simulink model "AUV_simulation_cmbined"  (R2024a)
settings: Solver=VariableStepAuto  StartTime=0.0  StopTime=10.0  RelTol=1e-3
model workspace (MAT data in the model file):
  T = 50
undefined symbols (not defined in the file): Acel_X, Acel_Y, Acel_Z, AUV, Cam_Left_Orientation, Cam_Left_Position, Cam_Right_Orientation, Cam_Right_Position, Gyro_X, Gyro_Y, Gyro_Z, Hydrophone_Bearing, Hydrophone_Distance, Leak_Detected, Pressure_Pa
libraries: nesl_utility x28, sm_lib x15, simulink x9
settings Model: Creator=adity  LastModifiedBy=adity

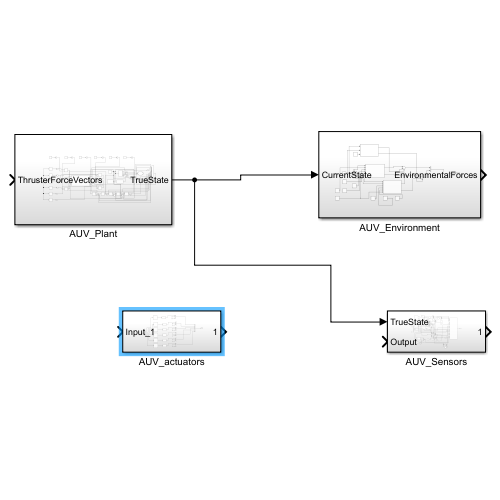
[thumbnail: Simulink's stored preview of the top-level diagram]
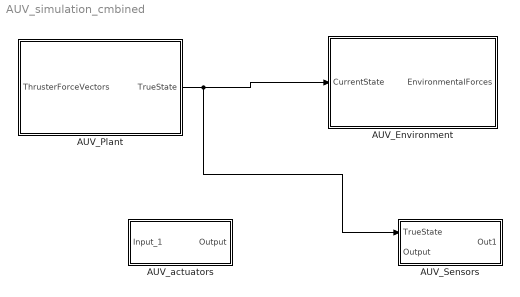
== system AUV_simulation_cmbined ==
  AUV_Environment : Subsystem
  AUV_Plant : Subsystem
  AUV_Sensors : Subsystem
  AUV_actuators : Subsystem
  wires:
  AUV_Plant/1(TrueState) -> AUV_Sensors/1(TrueState), AUV_Environment/1(CurrentState)

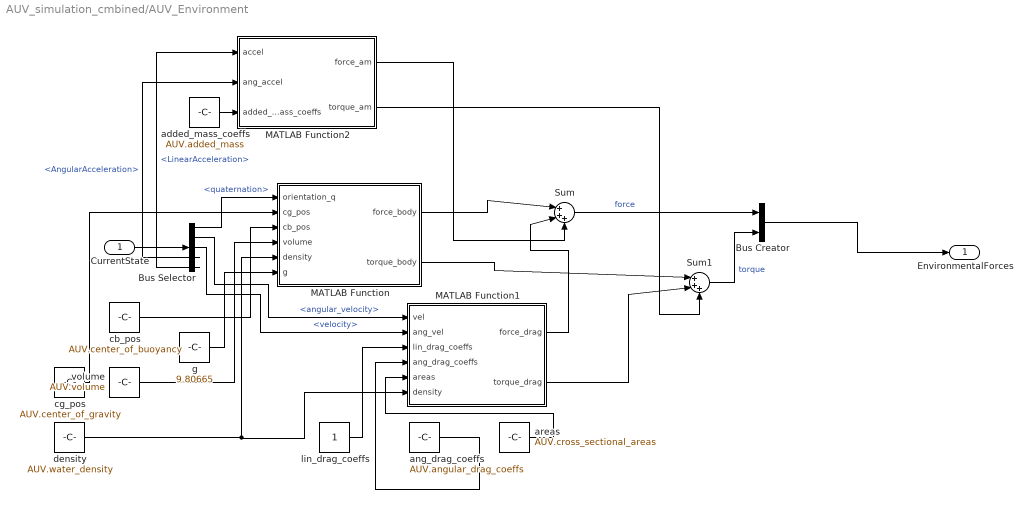
== system AUV_simulation_cmbined/AUV_Environment ==
  CurrentState : Inport
  Bus Creator : BusCreator  Inputs=2
  Bus Selector : BusSelector  OutputSignals=quaternation,angular_velocity,velocity,AngularAcceleration,LinearAcceleration
  MATLAB Function : MATLAB Function  TreatAsAtomicUnit=on
  MATLAB Function1 : MATLAB Function  TreatAsAtomicUnit=on
  MATLAB Function2 : MATLAB Function  TreatAsAtomicUnit=on
  Sum : Sum  Inputs=|+++
  Sum1 : Sum  Inputs=|+++
  added_mass_coeffs : Constant  Value=AUV.added_mass
  ang_drag_coeffs : Constant  Value=AUV.angular_drag_coeffs
  areas : Constant  Value=AUV.cross_sectional_areas
  cb_pos : Constant  Value=AUV.center_of_buoyancy
  cg_pos : Constant  Value=AUV.center_of_gravity
  density : Constant  Value=AUV.water_density
  g : Constant  Value=9.80665
  lin_drag_coeffs : Constant
  volume : Constant  Value=AUV.volume
  EnvironmentalForces : Outport
  wires:
  CurrentState/1 -> Bus Selector/1
  Bus Selector/1 -> MATLAB Function/1(orientation_q)  "<quaternation>"
  cg_pos/1 -> MATLAB Function/2(cg_pos)
  cb_pos/1 -> MATLAB Function/3(cb_pos)
  volume/1 -> MATLAB Function/4(volume)
  density/1 -> MATLAB Function/5(density), MATLAB Function1/6(density)
  g/1 -> MATLAB Function/6(g)
  Bus Selector/2 -> MATLAB Function1/1(vel)  "<angular_velocity>"
  Bus Selector/3 -> MATLAB Function1/2(ang_vel)  "<velocity>"
  areas/1 -> MATLAB Function1/5(areas)
  ang_drag_coeffs/1 -> MATLAB Function1/4(ang_drag_coeffs)
  lin_drag_coeffs/1 -> MATLAB Function1/3(lin_drag_coeffs)
  MATLAB Function/1(force_body) -> Sum/1
  MATLAB Function1/1(force_drag) -> Sum/2
  MATLAB Function/2(torque_body) -> Sum1/1
  MATLAB Function1/2(torque_drag) -> Sum1/2
  Sum/1 -> Bus Creator/1  "force"
  Sum1/1 -> Bus Creator/2  "torque"
  Bus Creator/1 -> EnvironmentalForces/1
  Bus Selector/4 -> MATLAB Function2/2(ang_accel)  "<AngularAcceleration>"
  Bus Selector/5 -> MATLAB Function2/1(accel)  "<LinearAcceleration>"
  added_mass_coeffs/1 -> MATLAB Function2/3(added_mass_coeffs)
  MATLAB Function2/2(torque_am) -> Sum1/3
  MATLAB Function2/1(force_am) -> Sum/3

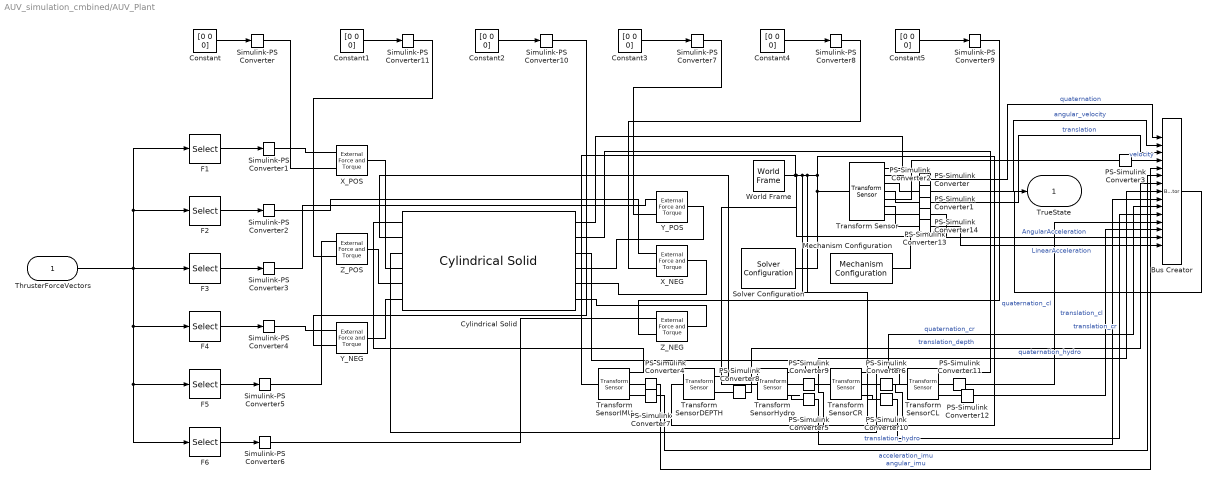
== system AUV_simulation_cmbined/AUV_Plant ==
  ThrusterForceVectors : Inport  PortDimensions=[6 3]
  Bus Creator : BusCreator  Inputs=15
  Constant{,1..5} (6 alike) : Constant  Value=[0 0 0]
  Cylindrical Solid : sm_lib/Body Elements/Cylindrical Solid  CylinderRadius=1  CylinderRadiusUnits=m  CylinderLength=1  CylinderLengthUnits=m  ExportEntireGeometry=off  InertiaType=Custom  BasedOnType=Density  Density=1000  DensityUnits=kg/m^3  Mass=AUV.mass  MassUnits=kg  CenterOfMass=AUV.center_of_gravity  CenterOfMassUnits=m  MomentsOfInertia=[AUV.inertia(1,1), AUV.inertia(2,2), AUV.inertia(3,3)]  MomentsOfInertiaUnits=kg*m^2  ProductsOfInertia=[AUV.inertia(2,3), AUV.inertia(1,3), AUV.inertia(1,2)]  ProductsOfInertiaUnits=kg*m^2  GraphicType=FromGeometry  MarkerShape=Sphere  MarkerSize=10  GraphicVisPropType=SimpleVisualProperties  GraphicDiffuseColor=[0.5 0.5 0.5]  GraphicOpacity=1  GraphicSpecularColor=[0.5 0.5 0.5 1.0]  GraphicAmbientColor=[0.15 0.15 0.15 1.0]  GraphicEmissiveColor=[0.0 0.0 0.0 1.0]  GraphicShininess=75  DoExposeReferenceFrame=on  SerializedFrames=<Frames><Frame><Id>Frame1</Id><Value><Name>IMU_Frame</Name><Origin><Source>ReferenceFrame</Source><FeatureName></FeatureName></Origin><PrimaryAxis><DefinedDirection>+Z</DefinedDirection><Source>ReferenceFrame</Source><SourceDirection>+Z</SourceDirection><FeatureName></FeatureName></PrimaryAxis><SecondaryAxis><DefinedDirection>+X</DefinedDirection><Source>ReferenceFrame</Source><SourceDirection>+X</SourceDirection><FeatureName></FeatureName></SecondaryAxis></Value></Frame><Frame><Id>Frame2</Id><Value><Name>DepthSensor_Frame</Name><Origin><Source>ReferenceFrame</Source><FeatureName></FeatureName></Origin><PrimaryAxis><DefinedDirection>+Z</DefinedDirection><Source>ReferenceFrame</Source><SourceDirection>+Z</SourceDirection><FeatureName></FeatureName></PrimaryAxis><SecondaryAxis><DefinedDirection>+X</DefinedDirection><Source>ReferenceFrame</Source><SourceDirection>+X</SourceDirection><FeatureName></FeatureName></SecondaryAxis></Value></Frame><Frame><Id>Frame3</Id><Value><Name>Camera_Left_Frame</Name><Origin><Source>ReferenceFrame</Source><FeatureName></FeatureName></Origin><PrimaryAxis><DefinedDirection>+Z</DefinedDirection><Source>ReferenceFrame</Source><SourceDirection>+Z</SourceDirection><FeatureName></FeatureName></PrimaryAxis><SecondaryAxis><DefinedDirection>+X</DefinedDirection><Source>ReferenceFrame</Source><SourceDirection>+X</SourceDirection><FeatureName></FeatureName></SecondaryAxis></Value></Frame><Frame><Id>Frame4</Id><Value><Name>Camera_Right_Frame</Name><Origin><Source>ReferenceFrame</Source><FeatureName></FeatureName></Origin><PrimaryAxis><DefinedDirection>+Z</DefinedDirection><Source>ReferenceFrame</Source><SourceDirection>+Z</SourceDirection><FeatureName></FeatureName></PrimaryAxis><SecondaryAxis><DefinedDirection>+X</DefinedDirection><Source>ReferenceFrame</Source><SourceDirection>+X</SourceDirection><FeatureName></FeatureName></SecondaryAxis></Value></Frame><Frame><Id>Frame5</Id><Value><Name>Hydrophone_Frame</Name><Origin><Source>ReferenceFrame</Source><FeatureName></FeatureName></Origin><PrimaryAxis><DefinedDirection>+Z</DefinedDirection><Source>ReferenceFrame</Source><SourceDirection>+Z</SourceDirection><FeatureName></FeatureName></PrimaryAxis><SecondaryAxis><DefinedDirection>+X</DefinedDirection><Source>ReferenceFrame</Source><SourceDirection>+X</SourceDirection><FeatureName></FeatureName></SecondaryAxis></Value></Frame><Frame><Id>Frame6</Id><Value><Name>Thruster_X_Pos</Name><Origin><Source>ReferenceFrame</Source><FeatureName></FeatureName></Origin><PrimaryAxis><DefinedDirection>+Z</DefinedDirection><Source>ReferenceFrame</Source><SourceDirection>+Z</SourceDirection><FeatureName></FeatureName></PrimaryAxis><SecondaryAxis><DefinedDirection>+X</DefinedDirection><Source>ReferenceFrame</Source><SourceDirection>+X</SourceDirection><FeatureName></FeatureName></SecondaryAxis></Value></Frame><Frame><Id>Frame7</Id><Value><Name>Thruster_Y_Pos</Name><Origin><Source>ReferenceFrame</Source><FeatureName></FeatureName></Origin><PrimaryAxis><DefinedDirection>+Z</DefinedDirection><Source>ReferenceFrame</Source><SourceDirection>+Z</SourceDirection><FeatureName></FeatureName></PrimaryAxis><SecondaryAxis><DefinedDirection>+X</DefinedDirection><Source>ReferenceFrame</Source><SourceDirection>+X</SourceDirection><FeatureName></FeatureName></SecondaryAxis></Value></Frame><Frame><Id>Frame8</Id><Value><Name>Thruster_Z_Pos</Name><Origin><Source>ReferenceFrame</Source><FeatureName></FeatureName></Origin><PrimaryAxis><DefinedDirection>+Z</DefinedDirection><Source>ReferenceFrame</Source><SourceDirection>+Z</SourceDirection><FeatureName></FeatureName></PrimaryAxis><SecondaryAxis><DefinedDirection>+X</DefinedDirection><Source>ReferenceFrame</Source><SourceDirection>+X</SourceDirection><FeatureName></FeatureName></SecondaryAxis></Value></Frame><Frame><Id>Frame9</Id><Value><Name>Thruster_X_Neg</Name><Origin><Source>ReferenceFrame</Source><FeatureName></FeatureName></Origin><PrimaryAxis><DefinedDirection>+Z</DefinedDirection><Source>ReferenceFrame</Source><SourceDirection>+Z</SourceDirection><FeatureName></FeatureName></PrimaryAxis><SecondaryAxis><DefinedDirection>+X</DefinedDirection><Source>ReferenceFrame</Source><SourceDirection>+X</SourceDirection><FeatureName></FeatureName></SecondaryAxis></Value></Frame><Frame><Id>Frame10</Id><Value><Name>Thruster_Y_Neg</Name><Origin><Source>ReferenceFrame</Source><FeatureName></FeatureName></Origin><PrimaryAxis><DefinedDirection>+Z</DefinedDirection><Source>ReferenceFrame</Source><SourceDirection>+Z</SourceDirection><FeatureName></FeatureName></PrimaryAxis><SecondaryAxis><DefinedDirection>+X</DefinedDirection><Source>ReferenceFrame</Source><SourceDirection>+X</SourceDirection><FeatureName></FeatureName></SecondaryAxis></Value></Frame><Frame><Id>Frame11</Id><Value><Name>Thruster_Z_Neg</Name><Origin><Source>ReferenceFrame</Source><FeatureName></FeatureName></Origin><PrimaryAxis><DefinedDirection>+Z</DefinedDirection><Source>ReferenceFrame</Source><SourceDirection>+Z</SourceDirection><FeatureName></FeatureName></PrimaryAxis><SecondaryAxis><DefinedDirection>+X</DefinedDirection><Source>ReferenceFrame</Source><SourceDirection>+X</SourceDirection><FeatureName></FeatureName></SecondaryAxis></Value></Frame></Frames>
  F1 : Selector  NumberOfDimensions=2  InputPortWidth=3  IndexOptions=Index vector (dialog),Select all  Indices=1,1  OutputSizes=1,1
  F2 : Selector  NumberOfDimensions=2  InputPortWidth=3  IndexOptions=Index vector (dialog),Select all  Indices=2,1  OutputSizes=1,1
  F3 : Selector  NumberOfDimensions=2  InputPortWidth=3  IndexOptions=Index vector (dialog),Select all  Indices=3,1  OutputSizes=1,1
  F4 : Selector  NumberOfDimensions=2  InputPortWidth=3  IndexOptions=Index vector (dialog),Select all  Indices=4,1  OutputSizes=1,1
  F5 : Selector  NumberOfDimensions=2  InputPortWidth=3  IndexOptions=Index vector (dialog),Select all  Indices=5,1  OutputSizes=1,1
  F6 : Selector  NumberOfDimensions=2  InputPortWidth=3  IndexOptions=Index vector (dialog),Select all  Indices=6,1  OutputSizes=1,1
  Mechanism Configuration : sm_lib/Utilities/Mechanism Configuration  UniformGravity=Constant  GravityVector=[0 0 9.80665]  GravityVectorUnits=m/s^2  LinearizationDelta=0.001  JointModeTransitionNonlinearIterations=2
  PS-Simulink Converter{,1..14} (15 alike) : nesl_utility/PS-Simulink Converter  PhysicalDomain=network_engine_domain  SubClassName=ps_output  LeftPortType=input  RightPortType=output  PseudoPeriodic=off  Frequencies=[]  VectorFormat=inherit  Unit=inherit  AffineConversion=off
  Simulink-PS Converter{,1..11} (12 alike) : nesl_utility/Simulink-PS Converter  PhysicalDomain=network_engine_domain  SubClassName=ps_input  LeftPortType=input  RightPortType=output  PseudoPeriodic=off  Frequencies=[]  NoiseDistribution=none  NoiseParameters=[]  Unit=1  AffineConversion=off  FilteringAndDerivatives=provide  SimscapeFilterOrder=1  InputFilterTimeConstant=0.001  UdotUserProvided=0
  Solver Configuration : nesl_utility/Solver Configuration  PhysicalDomain=network_engine_domain  SubClassName=solver  LeftPortType=input  RightPortType=generic  Tones=[]  Harmonics=[]  SimulateNoise=off  Profile=off  UseLocalSampling=off  EnableSwitchedLinearOptims=on  FrequencyDomain=off  UseCCode=off  RelTol=0.001  AbsTol=0.001  MinStep=1e-09  ToWorkspace=off  RevertToSquareIcSolve=off  NumHomotopyIterations=100  PhasorMode=off  PhasorModeNumHarmonics=1  ConsistencySolver=NEWTON_XTOL_AFTER_FTOL  IndexReductionMethod=DerivativeReplacement  DoDC=off  ResidualTolerance=1e-09  ConsistencyTolSource=GLOBAL  ConsistencyAbsTol=0.001  ConsistencyRelTol=0.001  ConsistencyTolFactor=0.001  UseLocalSolver=off  LocalSolverChoice=NE_BACKWARD_EULER_ADVANCER  ResolveIndetEquations=on  FunctionEvalNumThread=1  LocalSolverSampleTime=0.001  DoFixedCost=off  MaxNonlinIter=3  MaxModeIter=2  ComputeImpulses=off  ImpulseIterations=2  LinearAlgebra=auto  LinearAlgebraNumThread=0  EquationFormulation=NE_TIME_EF  DelaysMemoryBudget=1024  AutomaticFiltering=on  FilteringTimeConstant=0.001  PartitionStorageMethod=AS_NEEDED  PartitionMemoryBudget=1024  PartitionMethod=ROBUST  MultibodyUseLocalSolver=off  MultibodyLocalSolverChoice=ODE1  MultibodyLocalSolverSampleTime=0.001
  Transform Sensor : sm_lib/Frames and Transforms/Transform Sensor  MeasurementFrame=World  RotationSequence=XYX  SenseAngle=off  SenseAxis=off  SenseQ=on  SenseR=off  SenseRotationSequence=off  SenseOmegaX=off  SenseOmegaY=off  SenseOmegaZ=off  SenseOmega=on  SenseQDot=off  SenseRDot=off  SenseRotationSequenceDot=off  SenseAlphaX=off  SenseAlphaY=off  SenseAlphaZ=off  SenseAlpha=on  SenseQDDot=off  SenseRDDot=off  SenseX=off  SenseY=off  SenseZ=off  SenseXYZ=on  SenseRad=off  SenseAzim=off  SenseDist=off  SenseInc=off  SenseXDot=off  SenseYDot=off  SenseZDot=off  SenseXYZDot=on  SenseRadDot=off  SenseAzimDot=off  SenseDistDot=off  SenseIncDot=off  SenseXDDot=off  SenseYDDot=off  SenseZDDot=off  SenseXYZDDot=on  SenseRadDDot=off  SenseAzimDDot=off  SenseDistDDot=off  SenseIncDDot=off
  Transform SensorCL : sm_lib/Frames and Transforms/Transform Sensor  MeasurementFrame=World  RotationSequence=XYX  SenseAngle=off  SenseAxis=off  SenseQ=on  SenseR=off  SenseRotationSequence=off  SenseOmegaX=off  SenseOmegaY=off  SenseOmegaZ=off  SenseOmega=off  SenseQDot=off  SenseRDot=off  SenseRotationSequenceDot=off  SenseAlphaX=off  SenseAlphaY=off  SenseAlphaZ=off  SenseAlpha=off  SenseQDDot=off  SenseRDDot=off  SenseX=off  SenseY=off  SenseZ=off  SenseXYZ=on  SenseRad=off  SenseAzim=off  SenseDist=off  SenseInc=off  SenseXDot=off  SenseYDot=off  SenseZDot=off  SenseXYZDot=off  SenseRadDot=off  SenseAzimDot=off  SenseDistDot=off  SenseIncDot=off  SenseXDDot=off  SenseYDDot=off  SenseZDDot=off  SenseXYZDDot=off  SenseRadDDot=off  SenseAzimDDot=off  SenseDistDDot=off  SenseIncDDot=off
  Transform SensorCR : sm_lib/Frames and Transforms/Transform Sensor  MeasurementFrame=World  RotationSequence=XYX  SenseAngle=off  SenseAxis=off  SenseQ=on  SenseR=off  SenseRotationSequence=off  SenseOmegaX=off  SenseOmegaY=off  SenseOmegaZ=off  SenseOmega=off  SenseQDot=off  SenseRDot=off  SenseRotationSequenceDot=off  SenseAlphaX=off  SenseAlphaY=off  SenseAlphaZ=off  SenseAlpha=off  SenseQDDot=off  SenseRDDot=off  SenseX=off  SenseY=off  SenseZ=off  SenseXYZ=on  SenseRad=off  SenseAzim=off  SenseDist=off  SenseInc=off  SenseXDot=off  SenseYDot=off  SenseZDot=off  SenseXYZDot=off  SenseRadDot=off  SenseAzimDot=off  SenseDistDot=off  SenseIncDot=off  SenseXDDot=off  SenseYDDot=off  SenseZDDot=off  SenseXYZDDot=off  SenseRadDDot=off  SenseAzimDDot=off  SenseDistDDot=off  SenseIncDDot=off
  Transform SensorDEPTH : sm_lib/Frames and Transforms/Transform Sensor  MeasurementFrame=World  RotationSequence=XYX  SenseAngle=off  SenseAxis=off  SenseQ=off  SenseR=off  SenseRotationSequence=off  SenseOmegaX=off  SenseOmegaY=off  SenseOmegaZ=off  SenseOmega=off  SenseQDot=off  SenseRDot=off  SenseRotationSequenceDot=off  SenseAlphaX=off  SenseAlphaY=off  SenseAlphaZ=off  SenseAlpha=off  SenseQDDot=off  SenseRDDot=off  SenseX=off  SenseY=off  SenseZ=off  SenseXYZ=on  SenseRad=off  SenseAzim=off  SenseDist=off  SenseInc=off  SenseXDot=off  SenseYDot=off  SenseZDot=off  SenseXYZDot=off  SenseRadDot=off  SenseAzimDot=off  SenseDistDot=off  SenseIncDot=off  SenseXDDot=off  SenseYDDot=off  SenseZDDot=off  SenseXYZDDot=off  SenseRadDDot=off  SenseAzimDDot=off  SenseDistDDot=off  SenseIncDDot=off
  Transform SensorHydro : sm_lib/Frames and Transforms/Transform Sensor  MeasurementFrame=World  RotationSequence=XYX  SenseAngle=off  SenseAxis=off  SenseQ=on  SenseR=off  SenseRotationSequence=off  SenseOmegaX=off  SenseOmegaY=off  SenseOmegaZ=off  SenseOmega=off  SenseQDot=off  SenseRDot=off  SenseRotationSequenceDot=off  SenseAlphaX=off  SenseAlphaY=off  SenseAlphaZ=off  SenseAlpha=off  SenseQDDot=off  SenseRDDot=off  SenseX=off  SenseY=off  SenseZ=off  SenseXYZ=on  SenseRad=off  SenseAzim=off  SenseDist=off  SenseInc=off  SenseXDot=off  SenseYDot=off  SenseZDot=off  SenseXYZDot=off  SenseRadDot=off  SenseAzimDot=off  SenseDistDot=off  SenseIncDot=off  SenseXDDot=off  SenseYDDot=off  SenseZDDot=off  SenseXYZDDot=off  SenseRadDDot=off  SenseAzimDDot=off  SenseDistDDot=off  SenseIncDDot=off
  Transform SensorIMU : sm_lib/Frames and Transforms/Transform Sensor  MeasurementFrame=World  RotationSequence=XYX  SenseAngle=off  SenseAxis=off  SenseQ=off  SenseR=off  SenseRotationSequence=off  SenseOmegaX=off  SenseOmegaY=off  SenseOmegaZ=off  SenseOmega=on  SenseQDot=off  SenseRDot=off  SenseRotationSequenceDot=off  SenseAlphaX=off  SenseAlphaY=off  SenseAlphaZ=off  SenseAlpha=off  SenseQDDot=off  SenseRDDot=off  SenseX=off  SenseY=off  SenseZ=off  SenseXYZ=off  SenseRad=off  SenseAzim=off  SenseDist=off  SenseInc=off  SenseXDot=off  SenseYDot=off  SenseZDot=off  SenseXYZDot=off  SenseRadDot=off  SenseAzimDot=off  SenseDistDot=off  SenseIncDot=off  SenseXDDot=off  SenseYDDot=off  SenseZDDot=off  SenseXYZDDot=on  SenseRadDDot=off  SenseAzimDDot=off  SenseDistDDot=off  SenseIncDDot=off
  World Frame : sm_lib/Frames and Transforms/World Frame
  X_NEG : sm_lib/Forces and Torques/External Force and Torque  EnableForceX=off  EnableForceY=off  EnableForceZ=off  EnableForce=on  ForceResolutionFrame=AttachedFrame  EnableTorqueX=off  EnableTorqueY=off  EnableTorqueZ=off  EnableTorque=on  TorqueResolutionFrame=AttachedFrame
  X_POS : sm_lib/Forces and Torques/External Force and Torque  EnableForceX=off  EnableForceY=off  EnableForceZ=off  EnableForce=on  ForceResolutionFrame=AttachedFrame  EnableTorqueX=off  EnableTorqueY=off  EnableTorqueZ=off  EnableTorque=on  TorqueResolutionFrame=AttachedFrame
  Y_NEG : sm_lib/Forces and Torques/External Force and Torque  EnableForceX=off  EnableForceY=off  EnableForceZ=off  EnableForce=on  ForceResolutionFrame=AttachedFrame  EnableTorqueX=off  EnableTorqueY=off  EnableTorqueZ=off  EnableTorque=on  TorqueResolutionFrame=AttachedFrame
  Y_POS : sm_lib/Forces and Torques/External Force and Torque  EnableForceX=off  EnableForceY=off  EnableForceZ=off  EnableForce=on  ForceResolutionFrame=AttachedFrame  EnableTorqueX=off  EnableTorqueY=off  EnableTorqueZ=off  EnableTorque=on  TorqueResolutionFrame=AttachedFrame
  Z_NEG : sm_lib/Forces and Torques/External Force and Torque  EnableForceX=off  EnableForceY=off  EnableForceZ=off  EnableForce=on  ForceResolutionFrame=AttachedFrame  EnableTorqueX=off  EnableTorqueY=off  EnableTorqueZ=off  EnableTorque=on  TorqueResolutionFrame=AttachedFrame
  Z_POS : sm_lib/Forces and Torques/External Force and Torque  EnableForceX=off  EnableForceY=off  EnableForceZ=off  EnableForce=on  ForceResolutionFrame=AttachedFrame  EnableTorqueX=off  EnableTorqueY=off  EnableTorqueZ=off  EnableTorque=on  TorqueResolutionFrame=AttachedFrame
  TrueState : Outport
  wires:
  ThrusterForceVectors/1 -> F6/1, F5/1, F4/1, F3/1, F2/1, F1/1
  F1/1 -> Simulink-PS Converter1/1
  F2/1 -> Simulink-PS Converter2/1
  F3/1 -> Simulink-PS Converter3/1
  F4/1 -> Simulink-PS Converter4/1
  F5/1 -> Simulink-PS Converter5/1
  F6/1 -> Simulink-PS Converter6/1
  Constant/1 -> Simulink-PS Converter/1
  Constant1/1 -> Simulink-PS Converter11/1
  Constant2/1 -> Simulink-PS Converter10/1
  Constant3/1 -> Simulink-PS Converter7/1
  Constant4/1 -> Simulink-PS Converter8/1
  Constant5/1 -> Simulink-PS Converter9/1
  Bus Creator/1 -> TrueState/1
  PS-Simulink Converter/1 -> Bus Creator/1  "quaternation"
  PS-Simulink Converter2/1 -> Bus Creator/2  "angular_velocity"
  PS-Simulink Converter1/1 -> Bus Creator/3  "translation"
  PS-Simulink Converter3/1 -> Bus Creator/4  "velocity"
  PS-Simulink Converter4/1 -> Bus Creator/5  "angular_imu"
  PS-Simulink Converter7/1 -> Bus Creator/6  "acceleration_imu"
  PS-Simulink Converter8/1 -> Bus Creator/7  "translation_depth"
  PS-Simulink Converter9/1 -> Bus Creator/8  "quaternation_hydro"
  PS-Simulink Converter5/1 -> Bus Creator/9  "translation_hydro"
  PS-Simulink Converter6/1 -> Bus Creator/10  "quaternation_cr"
  PS-Simulink Converter10/1 -> Bus Creator/11  "translation_cr"
  PS-Simulink Converter11/1 -> Bus Creator/12  "quaternation_cl"
  PS-Simulink Converter12/1 -> Bus Creator/13  "translation_cl"
  PS-Simulink Converter14/1 -> Bus Creator/15  "LinearAcceleration"
  PS-Simulink Converter13/1 -> Bus Creator/14  "AngularAcceleration"
  connections:
  Cylindrical Solid/LConn4 -- X_POS/RConn1
  X_NEG/RConn1 -- Cylindrical Solid/RConn5
  Y_POS/RConn1 -- Cylindrical Solid/RConn4
  Z_NEG/RConn1 -- Cylindrical Solid/RConn6
  Y_NEG/RConn1 -- Cylindrical Solid/LConn6
  Z_POS/RConn1 -- Cylindrical Solid/LConn5
  Simulink-PS Converter1/RConn1 -- X_POS/LConn1
  Simulink-PS Converter2/RConn1 -- X_NEG/LConn1
  Simulink-PS Converter3/RConn1 -- Y_POS/LConn1
  Y_NEG/LConn1 -- Simulink-PS Converter4/RConn1
  Simulink-PS Converter5/RConn1 -- Z_POS/LConn1
  Simulink-PS Converter6/RConn1 -- Z_NEG/LConn1
  Simulink-PS Converter/RConn1 -- X_POS/LConn2
  Simulink-PS Converter11/RConn1 -- Z_POS/LConn2
  Simulink-PS Converter10/RConn1 -- Y_NEG/LConn2
  Simulink-PS Converter9/RConn1 -- Z_NEG/LConn2
  Simulink-PS Converter8/RConn1 -- X_NEG/LConn2
  Simulink-PS Converter7/RConn1 -- Y_POS/LConn2
  World Frame/RConn1 -- Transform SensorIMU/LConn1 -- Transform SensorHydro/LConn1 -- Mechanism Configuration/RConn1 -- Transform SensorDEPTH/LConn1 -- Transform SensorCL/LConn1 -- Transform SensorCR/LConn1 -- Solver Configuration/RConn1 -- Transform Sensor/LConn1
  Transform Sensor/RConn1 -- Cylindrical Solid/RConn1
  Transform Sensor/RConn2 -- PS-Simulink Converter/LConn1
  PS-Simulink Converter2/LConn1 -- Transform Sensor/RConn3
  PS-Simulink Converter1/LConn1 -- Transform Sensor/RConn4
  PS-Simulink Converter3/LConn1 -- Transform Sensor/RConn5
  Cylindrical Solid/LConn1 -- Transform SensorIMU/RConn1
  Transform SensorDEPTH/RConn1 -- Cylindrical Solid/LConn2
  Transform SensorHydro/RConn1 -- Cylindrical Solid/RConn3
  Cylindrical Solid/LConn3 -- Transform SensorCR/RConn1
  Transform SensorCL/RConn1 -- Cylindrical Solid/RConn2
  PS-Simulink Converter4/LConn1 -- Transform SensorIMU/RConn2
  PS-Simulink Converter7/LConn1 -- Transform SensorIMU/RConn3
  PS-Simulink Converter8/LConn1 -- Transform SensorDEPTH/RConn2
  PS-Simulink Converter6/LConn1 -- Transform SensorCR/RConn2
  Transform SensorHydro/RConn2 -- PS-Simulink Converter9/LConn1
  Transform SensorHydro/RConn3 -- PS-Simulink Converter5/LConn1
  PS-Simulink Converter10/LConn1 -- Transform SensorCR/RConn3
  PS-Simulink Converter12/LConn1 -- Transform SensorCL/RConn3
  PS-Simulink Converter11/LConn1 -- Transform SensorCL/RConn2
  PS-Simulink Converter13/LConn1 -- Transform Sensor/RConn6
  Transform Sensor/RConn7 -- PS-Simulink Converter14/LConn1

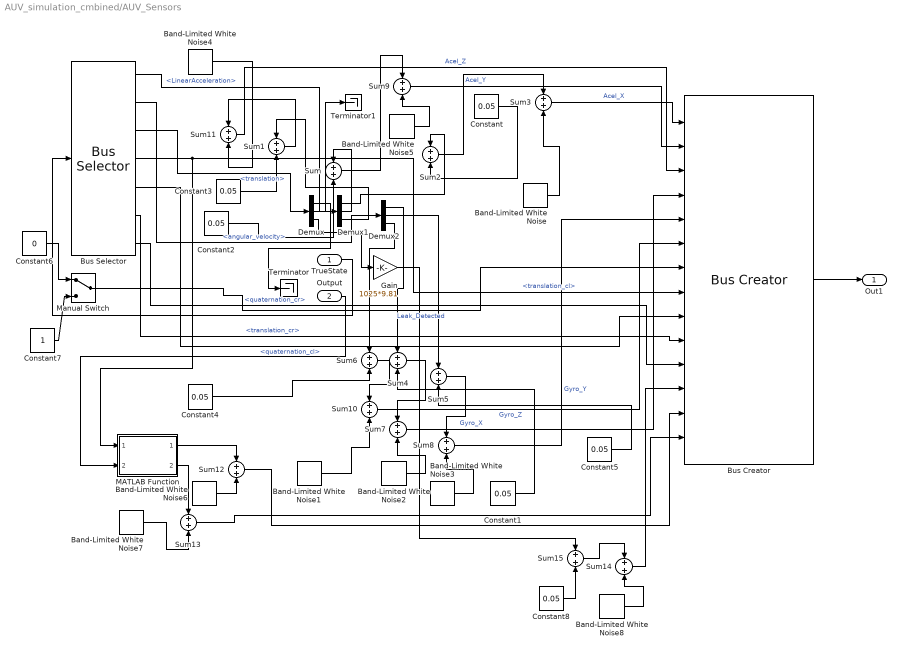
== system AUV_simulation_cmbined/AUV_Sensors ==
  TrueState : Inport
  Output : Inport  Port=2
  Band-Limited White Noise{,1..8} (9 alike) : simulink/Sources/Band-Limited White Noise  Cov=[0.1]  Ts=0.1  seed=[23341]
  Bus Creator : BusCreator  Inputs=Acel_X,Acel_Y,Acel_Z,Gyro_X,Gyro_Y,Gyro_Z,Leak_Detected,Cam_Left_Position,Cam_Left_Orientation,Cam_Right_Position,Cam_Right_Orientation,Pressure_Pa,Hydrophone_Distance,Hydrophone_Bearing
  Bus Selector : BusSelector  OutputSignals=LinearAcceleration,angular_velocity,translation,translation_cl,quaternation_cl,translation_cr,quaternation_cr
  Constant{,1..5,8} (7 alike) : Constant  Value=0.05
  Constant6 : Constant  Value=0
  Constant7 : Constant
  Demux : Demux  Outputs=3
  Demux1 : Demux  Outputs=3
  Demux2 : Demux  Outputs=3
  Gain : Gain  Gain=1025*9.81
  MATLAB Function : MATLAB Function  TreatAsAtomicUnit=on
  Manual Switch : ManualSwitch
  Sum{,1..15} (16 alike) : Sum
  Terminator : Terminator
  Terminator1 : Terminator
  Out1 : Outport
  wires:
  TrueState/1 -> Bus Selector/1
  Bus Creator/1 -> Out1/1
  Bus Selector/3 -> Demux/1  "<translation>"
  Bus Selector/1 -> Demux1/1  "<LinearAcceleration>"
  Bus Selector/2 -> Demux2/1  "<angular_velocity>"
  Demux/3 -> Gain/1
  Demux1/1 -> Sum2/1
  Constant/1 -> Sum2/2
  Sum2/1 -> Sum3/1
  Band-Limited White Noise/1 -> Sum3/2
  Demux1/2 -> Sum/1
  Demux1/3 -> Sum1/1
  Demux2/1 -> Sum4/1
  Demux2/2 -> Sum5/1
  Demux2/3 -> Sum6/1
  Constant4/1 -> Sum6/2
  Constant3/1 -> Sum1/2
  Constant2/1 -> Sum/2
  Constant1/1 -> Sum4/2
  Constant5/1 -> Sum5/2
  Sum1/1 -> Sum11/1
  Sum/1 -> Sum9/1
  Sum6/1 -> Sum10/1
  Sum4/1 -> Sum7/1
  Sum5/1 -> Sum8/1
  Band-Limited White Noise1/1 -> Sum10/2
  Band-Limited White Noise2/1 -> Sum7/2
  Band-Limited White Noise3/1 -> Sum8/2
  Band-Limited White Noise4/1 -> Sum11/2
  Band-Limited White Noise5/1 -> Sum9/2
  Sum3/1 -> Bus Creator/1  "Acel_X"
  Sum9/1 -> Bus Creator/2  "Acel_Y"
  Sum11/1 -> Bus Creator/3  "Acel_Z"
  Sum7/1 -> Bus Creator/4  "Gyro_X"
  Sum8/1 -> Bus Creator/5  "Gyro_Y"
  Sum10/1 -> Bus Creator/6  "Gyro_Z"
  Constant6/1 -> Manual Switch/1
  Constant7/1 -> Manual Switch/2
  Manual Switch/1 -> Bus Creator/7  "Leak_Detected"
  Bus Selector/4 -> Bus Creator/8, MATLAB Function/1(auv_pos)  "<translation_cl>"
  Bus Selector/5 -> Bus Creator/9  "<quaternation_cl>"
  Bus Selector/6 -> Bus Creator/10  "<translation_cr>"
  Bus Selector/7 -> Bus Creator/11  "<quaternation_cr>"
  Output/1 -> MATLAB Function/2(beacon_pos)
  MATLAB Function/1(distance) -> Sum12/1
  Band-Limited White Noise6/1 -> Sum12/2
  Band-Limited White Noise7/1 -> Sum13/2
  MATLAB Function/2(bearing) -> Sum13/1
  Sum12/1 -> Bus Creator/13
  Sum13/1 -> Bus Creator/14
  Gain/1 -> Sum15/1
  Constant8/1 -> Sum15/2
  Sum15/1 -> Sum14/1
  Band-Limited White Noise8/1 -> Sum14/2
  Sum14/1 -> Bus Creator/12
  Demux/1 -> Terminator/1
  Demux/2 -> Terminator1/1

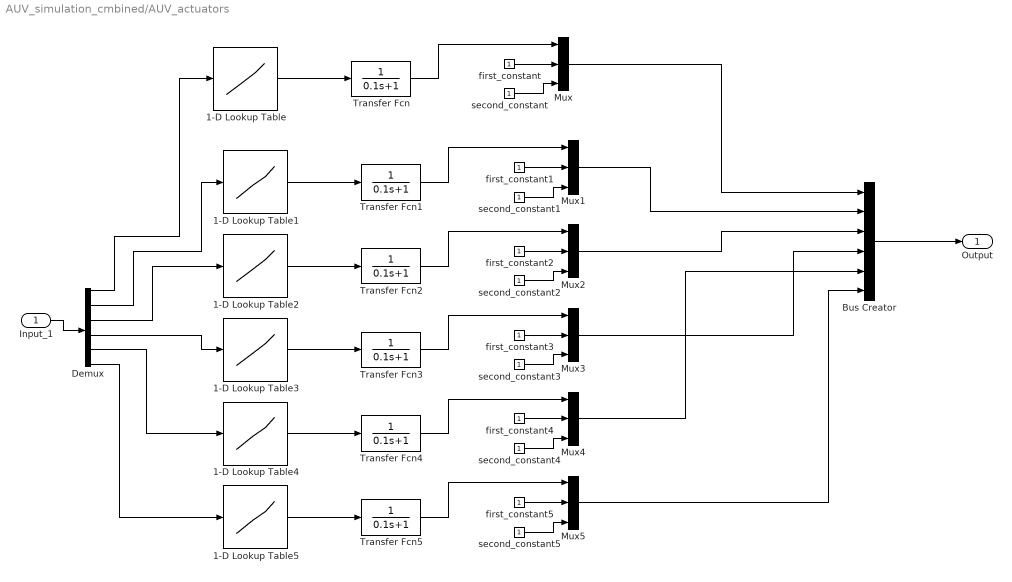
== system AUV_simulation_cmbined/AUV_actuators ==
  Input_1 : Inport
  1-D Lookup Table{,1..5} (6 alike) : Lookup_n-D  NumberOfTableDimensions=1  BreakpointsForDimension1=[-1,-0.1,0,0.1,1]  Table=[-40,-1,0,1,50]  InternalRulePriority=Speed  RndMeth=Simplest
  Bus Creator : BusCreator  Inputs=6
  Demux : Demux  Outputs=6
  Mux{,1..5} (6 alike) : Mux  Inputs=3
  Transfer Fcn{,1..5} (6 alike) : TransferFcn  Denominator=[0.1 1]
  first_constant{,1..5} (6 alike) : Constant
  second_constant{,1..5} (6 alike) : Constant
  Output : Outport
  wires:
  Demux/1 -> 1-D Lookup Table/1
  1-D Lookup Table/1 -> Transfer Fcn/1
  Transfer Fcn/1 -> Mux/1
  first_constant/1 -> Mux/2
  second_constant/1 -> Mux/3
  first_constant1/1 -> Mux1/2
  1-D Lookup Table1/1 -> Transfer Fcn1/1
  second_constant1/1 -> Mux1/3
  Demux/2 -> 1-D Lookup Table1/1
  Transfer Fcn1/1 -> Mux1/1
  Transfer Fcn2/1 -> Mux2/1
  second_constant2/1 -> Mux2/3
  first_constant2/1 -> Mux2/2
  1-D Lookup Table2/1 -> Transfer Fcn2/1
  Demux/3 -> 1-D Lookup Table2/1
  Transfer Fcn3/1 -> Mux3/1
  second_constant3/1 -> Mux3/3
  first_constant3/1 -> Mux3/2
  1-D Lookup Table3/1 -> Transfer Fcn3/1
  Demux/4 -> 1-D Lookup Table3/1
  Transfer Fcn4/1 -> Mux4/1
  second_constant4/1 -> Mux4/3
  first_constant4/1 -> Mux4/2
  1-D Lookup Table4/1 -> Transfer Fcn4/1
  Demux/5 -> 1-D Lookup Table4/1
  Transfer Fcn5/1 -> Mux5/1
  second_constant5/1 -> Mux5/3
  first_constant5/1 -> Mux5/2
  1-D Lookup Table5/1 -> Transfer Fcn5/1
  Demux/6 -> 1-D Lookup Table5/1
  Mux/1 -> Bus Creator/1
  Mux1/1 -> Bus Creator/2
  Mux2/1 -> Bus Creator/3
  Mux3/1 -> Bus Creator/4
  Mux4/1 -> Bus Creator/5
  Mux5/1 -> Bus Creator/6
  Input_1/1 -> Demux/1
  Bus Creator/1 -> Output/1

== matlab function AUV_simulation_cmbined/AUV_Environment/MATLAB Function1 ==
  data: vel input; force_drag output; ang_vel input; lin_drag_coeffs input; ang_drag_coeffs input; areas input; density input; torque_drag output
function [force_drag, torque_drag] = drag_model(vel, ang_vel, lin_drag_coeffs, ang_drag_coeffs, areas, density)
    % Calculates hydrodynamic drag forces and torques in the body frame
    % vel:      Linear velocity vector [vx, vy, vz]
    % ang_vel:  Angular velocity vector [p, q, r]

    % --- Linear Drag ---
    % Using the quadratic drag formula: Fd = -0.5 * rho * v^2 * Cd * A
    % The sign() function ensures the force always opposes the velocity.
    force_drag = -sign(vel) .* (0.5 * density .* (vel.^2) .* lin_drag_coeffs .* areas);

    % --- Angular Drag (Rotational Resistance) ---
    % A similar model for rotational drag. We use a length^5 term for scaling,
    % assuming a characteristic length of 1m for simplicity.
    torque_drag = -sign(ang_vel) .* (0.5 * density .* (ang_vel.^2) .* ang_drag_coeffs);
endfunction y = fcn(u)

y = u;

== matlab function AUV_simulation_cmbined/AUV_Environment/MATLAB Function ==
  data: orientation_q input; force_body output; cg_pos input; cb_pos input; volume input; density input; g input; torque_body output
function [force_body, torque_body] = buoyancy_model(orientation_q, cg_pos, cb_pos, volume, density, g)
    % This function calculates buoyancy force and torque in the AUV's body frame.
    % orientation_q: quaternion [w, x, y, z] from the plant
    % cg_pos: Center of Gravity position vector [x, y, z] in body frame
    % cb_pos: Center of Buoyancy position vector [x, y, z] in body frame

    % 1. Calculate the buoyant force vector in the world frame (upward)
    force_magnitude = volume * density * g;
    force_world = [0; 0; -force_magnitude]; % Upward force in our Z-down world

    % 2. Rotate the world force vector into the AUV's body frame
    % We use the inverse of the AUV's orientation to rotate a world vector to body
    force_body = quatrotate(quatinv(orientation_q), force_world')';

    % 3. Calculate the torque produced by this force acting at the Center of Buoyancy
    % Torque = r x F, where r is the vector from the CG to the CB
    lever_arm = cb_pos - cg_pos;
    torque_body = cross(lever_arm, force_body);
end

== matlab function AUV_simulation_cmbined/AUV_Environment/MATLAB Function2 ==
  data: accel input; force_am output; ang_accel input; added_mass_coeffs input; torque_am output
function [force_am, torque_am] = added_mass_model(accel, ang_accel, added_mass_coeffs)
    % Calculates the forces and torques due to added mass.
    % F = -m_added * acceleration

    % Split the 6-element coeff vector into linear and angular parts
    added_mass_linear = added_mass_coeffs(1:3);
    added_mass_angular = added_mass_coeffs(4:6);

    force_am = -added_mass_linear .* accel;
    torque_am = -added_mass_angular .* ang_accel;
end

== matlab function AUV_simulation_cmbined/AUV_Sensors/MATLAB Function ==
  data: auv_pos input; distance output; beacon_pos input; bearing output
function [distance, bearing] = fcn(auv_pos, beacon_pos)
% This function calculates the distance and bearing from the AUV to a beacon.

% Calculate the vector from the AUV to the beacon
vector_to_beacon = beacon_pos - auv_pos;

% Calculate the 3D distance (magnitude of the vector)
distance = sqrt(vector_to_beacon(1)^2 + vector_to_beacon(2)^2 + vector_to_beacon(3)^2);

% Calculate the bearing (the angle in the horizontal X-Y plane)
% atan2 is used to get the correct angle from -pi to +pi
bearing = atan2(vector_to_beacon(2), vector_to_beacon(1));

end
